simulink library "Estimator"  (R2014b)
settings: Solver=ode45  StartTime=0.0  StopTime=10.0  RelTol=1e-3
undefined symbols (not defined in the file): ConfParam
libraries: Qinverse x1, Qprod x1, Quat2Rot x1
settings Model: Creator=Hp  LastModifiedBy=Hp

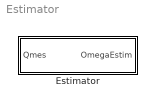
== system Estimator ==
  Estimator : Subsystem

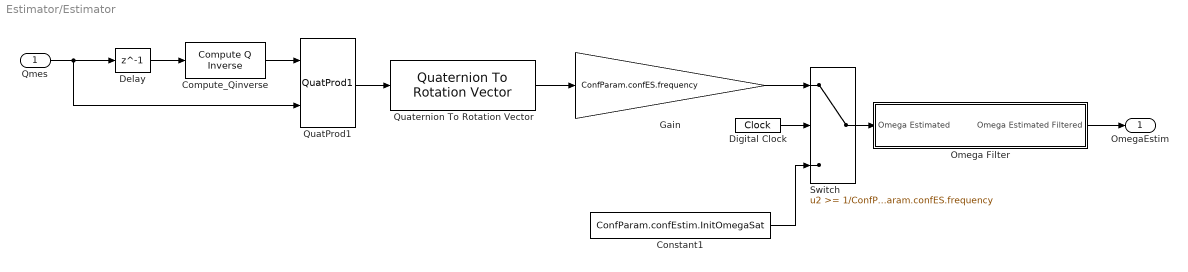
== system Estimator/Estimator ==
  Qmes : Inport
  Compute_Qinverse : Qinverse/Compute Q Inverse
  Constant1 : Constant  Value=ConfParam.confEstim.InitOmegaSat
  Delay : Delay  DelayLength=1  InitialCondition=ConfParam.confEstim.InitQsat  SampleTime=1/ConfParam.confES.frequency
  Digital Clock : DigitalClock  SampleTime=1/ConfParam.confES.frequency
  Gain : Gain  Gain=ConfParam.confES.frequency
  Omega Filter : Subsystem
  QuatProd1 : Qprod/QuatProd1
  Quaternion To Rotation Vector : Quat2Rot/Quaternion To Rotation Vector
  Switch : Switch  Threshold=1/ConfParam.confES.frequency  SampleTime=1/ConfParam.confES.frequency
  OmegaEstim : Outport
  wires:
  Delay/1 -> Compute_Qinverse/1
  Quaternion To Rotation Vector/1 -> Gain/1
  Gain/1 -> Switch/1
  Compute_Qinverse/1 -> QuatProd1/1
  QuatProd1/1 -> Quaternion To Rotation Vector/1
  Digital Clock/1 -> Switch/2
  Switch/1 -> Omega Filter/1(Omega Estimated)
  Constant1/1 -> Switch/3
  Qmes/1 -> QuatProd1/2, Delay/1
  Omega Filter/1(Omega Estimated Filtered) -> OmegaEstim/1

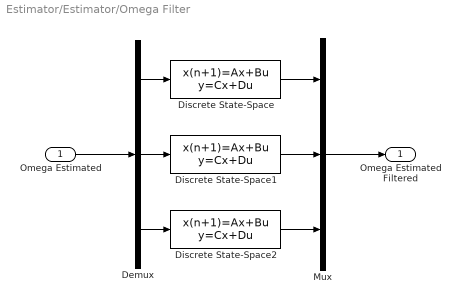
== system Estimator/Estimator/Omega Filter ==
  Omega Estimated : Inport
  Demux : Demux  Outputs=3
  Discrete State-Space : DiscreteStateSpace  A=ConfParam.confEstim.V_A  B=ConfParam.confEstim.V_B  C=ConfParam.confEstim.V_C  D=ConfParam.confEstim.V_D  X0=[ConfParam.confEstim.InitOmegaSat(1)/ConfParam.confEstim.V_OmegaN^2; 0]  SampleTime=1/ConfParam.confES.frequency
  Discrete State-Space1 : DiscreteStateSpace  A=ConfParam.confEstim.V_A  B=ConfParam.confEstim.V_B  C=ConfParam.confEstim.V_C  D=ConfParam.confEstim.V_D  X0=[ConfParam.confEstim.InitOmegaSat(2)/ConfParam.confEstim.V_OmegaN^2; 0]  SampleTime=1/ConfParam.confES.frequency
  Discrete State-Space2 : DiscreteStateSpace  A=ConfParam.confEstim.V_A  B=ConfParam.confEstim.V_B  C=ConfParam.confEstim.V_C  D=ConfParam.confEstim.V_D  X0=[ConfParam.confEstim.InitOmegaSat(3)/ConfParam.confEstim.V_OmegaN^2; 0]  SampleTime=1/ConfParam.confES.frequency
  Mux : Mux  Inputs=3
  Omega Estimated Filtered : Outport
  wires:
  Mux/1 -> Omega Estimated Filtered/1
  Discrete State-Space/1 -> Mux/1
  Discrete State-Space1/1 -> Mux/2
  Discrete State-Space2/1 -> Mux/3
  Omega Estimated/1 -> Demux/1
  Demux/1 -> Discrete State-Space/1
  Demux/2 -> Discrete State-Space1/1
  Demux/3 -> Discrete State-Space2/1
